simulink model "PV_module_model"  (R2022b)
settings: Solver=VariableStepAuto  StartTime=0.0  StopTime=1  FixedStep=10e-6  RelTol=1e-3
undefined symbols (not defined in the file): sigbuilder_block
libraries: slpidlib x1
settings Model: Creator=amahe  LastModifiedBy=amahe

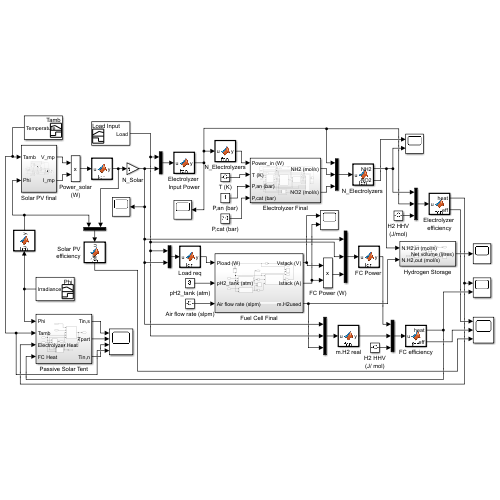
[thumbnail: Simulink's stored preview of the top-level diagram]
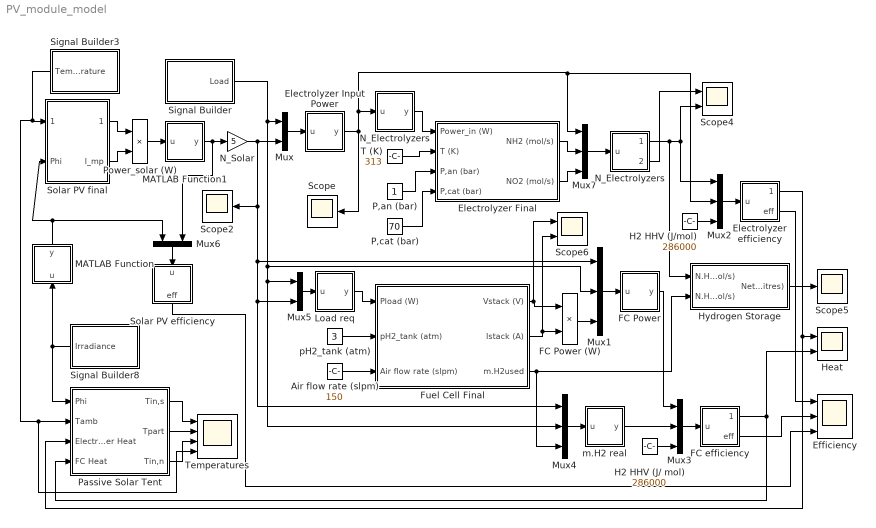
== system PV_module_model ==
  Air flow rate (slpm) : Constant  Value=150
  Efficiency : Scope  NumInputPorts=3
  Electrolyzer Input Power : MATLAB Function  TreatAsAtomicUnit=on
  Electrolyzer efficiency : MATLAB Function  TreatAsAtomicUnit=on
  Electrolyzer Final : Subsystem
  "FC Power " : MATLAB Function  TreatAsAtomicUnit=on
  FC Power (W) : Product
  FC efficiency : MATLAB Function  TreatAsAtomicUnit=on
  Fuel Cell Final : Subsystem
  H2 HHV (J/ mol) : Constant  Value=286000
  H2 HHV (J/mol) : Constant  Value=286000
  Heat : Scope  NumInputPorts=2
  Hydrogen Storage : Subsystem
  Load req : MATLAB Function  TreatAsAtomicUnit=on
  MATLAB Function : MATLAB Function  TreatAsAtomicUnit=on
  MATLAB Function1 : MATLAB Function  TreatAsAtomicUnit=on
  Mux : Mux  Inputs=2
  Mux{1..4,7} (5 alike) : Mux  Inputs=3
  Mux5 : Mux  Inputs=2
  Mux6 : Mux  Inputs=2
  N_Electrolyzers : MATLAB Function  TreatAsAtomicUnit=on
  "N_Electrolyzers " : MATLAB Function  TreatAsAtomicUnit=on
  N_Solar : Gain  Gain=5
  P,an (bar) : Constant
  P,cat (bar) : Constant  Value=70
  Passive Solar Tent : Subsystem
  Power_solar (W) : Product
  Scope : Scope
  Scope2 : Scope
  Scope4 : Scope  NumInputPorts=2
  Scope5 : Scope
  Scope6 : Scope  NumInputPorts=2
  Signal Builder : Subsystem  Tag=STV Subsys  LoadFcn=sigbuilder_block('load');  StartFcn=sigbuilder_block('start');  StopFcn=sigbuilder_block('stop');  ClipboardFcn=sigbuilder_block('clipboard');  mask(Sigbuilder block){tuvar=[0:10]}
      mask help: Simulink:masks:SigbuilderBlock_MD
      mask init:
      | if ~strcmp(get_param(bdroot(gcbh),'SimulationStatus'),'stopped') tuvar = sigbuilder_block('maskInit'); end
      settings: CopyFcn=sigbuilder_block('copy');  DeleteFcn=sigbuilder_block('delete');  ModelCloseFcn=sigbuilder_block('modelClose');  PreSaveFcn=sigbuilder_block('preSave');  PauseFcn=sigbuilder_block('pause');  ContinueFcn=sigbuilder_block('continue');  NameChangeFcn=sigbuilder_block('namechange');  OpenFcn=sigbuilder_block('open',[425.4 150.6 550.8 400.2 ]);  CloseFcn=sigbuilder_block('close');
      mask Display: plot(0, 0, 100, 100,[2, 2, 32, 32, 2], [68, 8, 8, 68, 68],[32, 2], [38, 38], [32, 19, 2],[53, 60, 44], [32, 17, 17, 2],[16, 16, 31, 31]);txt = getActiveGroup(gcbh);text(2, 100, txt,'verticalAlignment', 'top');
  Signal Builder3 : Subsystem  Tag=STV Subsys  LoadFcn=sigbuilder_block('load');  StartFcn=sigbuilder_block('start');  StopFcn=sigbuilder_block('stop');  ClipboardFcn=sigbuilder_block('clipboard');  mask(Sigbuilder block){tuvar=[0:10]}
      mask help: Simulink:masks:SigbuilderBlock_MD
      mask init:
      | if ~strcmp(get_param(bdroot(gcbh),'SimulationStatus'),'stopped') tuvar = sigbuilder_block('maskInit'); end
      settings: CopyFcn=sigbuilder_block('copy');  DeleteFcn=sigbuilder_block('delete');  ModelCloseFcn=sigbuilder_block('modelClose');  PreSaveFcn=sigbuilder_block('preSave');  PauseFcn=sigbuilder_block('pause');  ContinueFcn=sigbuilder_block('continue');  NameChangeFcn=sigbuilder_block('namechange');  OpenFcn=sigbuilder_block('open',[437.6 199.2 550.4 400 ]);  CloseFcn=sigbuilder_block('close');
      mask Display: plot(0, 0, 100, 100,[2, 2, 32, 32, 2], [68, 8, 8, 68, 68],[32, 2], [38, 38], [32, 19, 2],[53, 60, 44], [32, 17, 17, 2],[16, 16, 31, 31]);txt = getActiveGroup(gcbh);text(2, 100, txt,'verticalAlignment', 'top');
  Signal Builder8 : Subsystem  Tag=STV Subsys  LoadFcn=sigbuilder_block('load');  StartFcn=sigbuilder_block('start');  StopFcn=sigbuilder_block('stop');  ClipboardFcn=sigbuilder_block('clipboard');  mask(Sigbuilder block){tuvar=[0:10]}
      mask help: Simulink:masks:SigbuilderBlock_MD
      mask init:
      | if ~strcmp(get_param(bdroot(gcbh),'SimulationStatus'),'stopped') tuvar = sigbuilder_block('maskInit'); end
      settings: CopyFcn=sigbuilder_block('copy');  DeleteFcn=sigbuilder_block('delete');  ModelCloseFcn=sigbuilder_block('modelClose');  PreSaveFcn=sigbuilder_block('preSave');  PauseFcn=sigbuilder_block('pause');  ContinueFcn=sigbuilder_block('continue');  NameChangeFcn=sigbuilder_block('namechange');  OpenFcn=sigbuilder_block('open',[437.6 199.2 550.4 400 ]);  CloseFcn=sigbuilder_block('close');
      mask Display: plot(0, 0, 100, 100,[2, 2, 32, 32, 2], [68, 8, 8, 68, 68],[32, 2], [38, 38], [32, 19, 2],[53, 60, 44], [32, 17, 17, 2],[16, 16, 31, 31]);txt = getActiveGroup(gcbh);text(2, 100, txt,'verticalAlignment', 'top');
  Solar PV efficiency : MATLAB Function  TreatAsAtomicUnit=on
  Solar PV final : Subsystem
  T (K) : Constant  Value=313
  Temperatures : Scope  NumInputPorts=4
  m.H2 real : MATLAB Function  TreatAsAtomicUnit=on
  pH2_tank (atm) : Constant  Value=3
  wires:
  Electrolyzer Final/2(NO2 (mol/s)) -> Mux7/3
  Passive Solar Tent/1(Tin,s) -> Temperatures/1
  Mux7/1 -> "N_Electrolyzers "/1(u)
  Power_solar (W)/1 -> MATLAB Function1/1(u)
  "N_Electrolyzers "/1(NH2) -> Hydrogen Storage/1(N.H2,in (mol/s)), Mux2/1, Scope4/2
  FC efficiency/1(heat) -> Passive Solar Tent/4(FC Heat), Heat/2
  FC efficiency/2(eff) -> Efficiency/2
  Mux/1 -> Electrolyzer Input Power/1(u)
  P,cat (bar)/1 -> Electrolyzer Final/4(P,cat (bar))
  Mux6/1 -> Solar PV efficiency/1(u)
  Signal Builder3/1(Temperature) -> Passive Solar Tent/2(Tamb), Temperatures/4, Solar PV final/1(Tamb)
  Electrolyzer efficiency/1(heat) -> Passive Solar Tent/3(Electrolyzer Heat), Heat/1
  Air flow rate (slpm)/1 -> Fuel Cell Final/3(Air flow rate (slpm))
  m.H2 real/1(y) -> Mux3/2
  Electrolyzer efficiency/2(eff) -> Efficiency/1
  "N_Electrolyzers "/2(NO2) -> Scope4/1
  Hydrogen Storage/1(Net volume (litres)) -> Scope5/1
  Passive Solar Tent/2(Tpart) -> Temperatures/2
  Electrolyzer Input Power/1(y) -> Mux2/2, Mux7/1, N_Electrolyzers/1(u), Scope/1
  Mux3/1 -> FC efficiency/1(u)
  MATLAB Function/1(y) -> Mux6/1, Solar PV final/2(Phi)
  T (K)/1 -> Electrolyzer Final/2(T (K))
  FC Power (W)/1 -> Mux1/3
  Solar PV final/2(I_mp) -> Power_solar (W)/2
  Fuel Cell Final/2(Istack (A)) -> Scope6/2, FC Power (W)/2
  Fuel Cell Final/3(m.H2used) -> Mux4/3, Hydrogen Storage/2(N.H2,out (mol/s))
  Electrolyzer Final/1(NH2 (mol/s)) -> Mux7/2
  Passive Solar Tent/3(Tin,n) -> Temperatures/3
  Fuel Cell Final/1(Vstack (V)) -> Scope6/1, FC Power (W)/1
  MATLAB Function1/1(y) -> N_Solar/1, Mux6/2
  Mux2/1 -> Electrolyzer efficiency/1(u)
  Solar PV efficiency/1(eff) -> Efficiency/3
  Signal Builder/1(Load) -> Mux4/2, Mux5/1, Mux1/2, Mux/1
  P,an (bar)/1 -> Electrolyzer Final/3(P,an (bar))
  Mux1/1 -> "FC Power "/1(u)
  Signal Builder8/1(Irradiance) -> Passive Solar Tent/1(Phi), MATLAB Function/1(u)
  H2 HHV (J/ mol)/1 -> Mux3/3
  "FC Power "/1(y) -> Mux3/1
  pH2_tank (atm)/1 -> Fuel Cell Final/2(pH2_tank (atm))
  H2 HHV (J/mol)/1 -> Mux2/3
  Mux5/1 -> Load req/1(u)
  N_Electrolyzers/1(y) -> Electrolyzer Final/1(Power_in (W))
  Solar PV final/1(V_mp) -> Power_solar (W)/1
  Load req/1(y) -> Fuel Cell Final/1(Pload (W))
  N_Solar/1 -> Mux/2, Mux1/1, Mux4/1, Mux5/2, Scope2/1
  Mux4/1 -> m.H2 real/1(u)

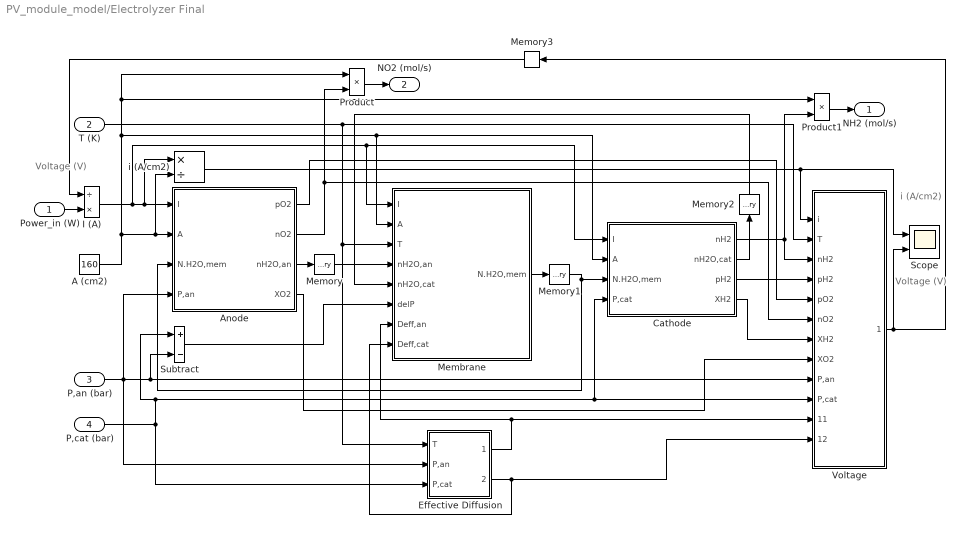
== system PV_module_model/Electrolyzer Final ==
  note: Voltage (V)
  note: i (A/cm2)
  note: Voltage
      | (V)
  Power_in (W) : Inport
  T (K) : Inport  Port=2
  P,an (bar) : Inport  Port=3
  P,cat (bar) : Inport  Port=4
  A (cm2) : Constant  Value=160
  Anode : Subsystem
  Cathode : Subsystem
  Effective Diffusion : Subsystem
  I (A) : Product  Inputs=/*
  Membrane : Subsystem
  Memory : Memory  InitialCondition=10^6
  Memory1 : Memory  InitialCondition=1
  Memory2 : Memory  InitialCondition=10^6
  Memory3 : Memory  InitialCondition=2
  Product : Product  Inputs=**
  Product1 : Product  Inputs=**
  Scope : Scope  NumInputPorts=2
  Subtract : Sum  Inputs=+-
  Voltage : Subsystem
  i (A/cm2) : Product  Inputs=*/
  NH2 (mol/s) : Outport
  NO2 (mol/s) : Outport  Port=2
  wires:
  A (cm2)/1 -> i (A/cm2)/2, Anode/2(A), Product/1, Product1/1, Cathode/2(A), Membrane/2(A)
  I (A)/1 -> Membrane/1(I), Cathode/1(I), i (A/cm2)/1, Anode/1(I)
  Cathode/3(pH2) -> Voltage/4(pH2)
  Membrane/1(N.H2O,mem) -> Memory1/1
  P,cat (bar)/1 -> Effective Diffusion/3(P,cat), Subtract/1, Cathode/4(P,cat), Voltage/10(P,cat)
  Anode/3(nH2O,an) -> Memory/1
  i (A/cm2)/1 -> Scope/1, Voltage/1(i)
  Memory/1 -> Membrane/4(nH2O,an)
  Anode/4(XO2) -> Voltage/8(XO2)
  Effective Diffusion/1(Deff,an) -> Voltage/11(Deff,an), Membrane/7(Deff,an)
  Voltage/1(Voltage (V)) -> Memory3/1, Scope/2
  Power_in (W)/1 -> I (A)/2
  T (K)/1 -> Membrane/3(T), Effective Diffusion/1(T), Voltage/2(T)
  Cathode/2(nH2O,cat) -> Memory2/1
  Memory1/1 -> Anode/3(N.H2O,mem), Cathode/3(N.H2O,mem)
  Memory2/1 -> Membrane/5(nH2O,cat)
  Memory3/1 -> I (A)/1
  Product/1 -> NO2 (mol/s)/1
  Effective Diffusion/2(Deff,cat) -> Voltage/12(Deff,cat), Membrane/8(Deff,cat)
  Cathode/4(XH2) -> Voltage/7(XH2)
  Cathode/1(nH2) -> Product1/2, Voltage/3(nH2)
  Subtract/1 -> Membrane/6(delP)
  Product1/1 -> NH2 (mol/s)/1
  Anode/1(pO2) -> Voltage/5(pO2)
  P,an (bar)/1 -> Anode/4(P,an), Effective Diffusion/2(P,an), Subtract/2, Voltage/9(P,an)
  Anode/2(nO2) -> Product/2, Voltage/6(nO2)

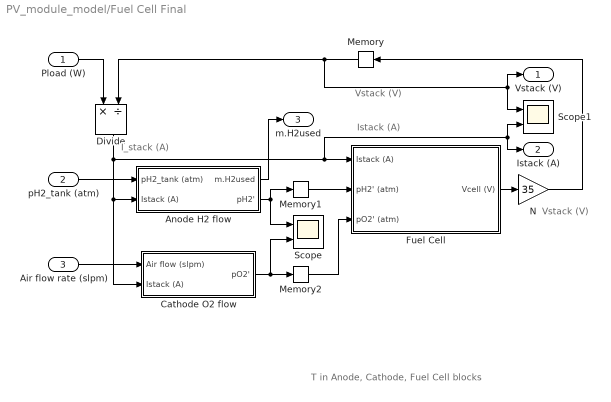
== system PV_module_model/Fuel Cell Final ==
  note: T in Anode, Cathode, Fuel Cell blocks
  note: I_stack (A)
  note: Vstack (V)
  note: Istack (A)
  note: Vstack (V)
  Pload (W) : Inport
  pH2_tank (atm) : Inport  Port=2
  Air flow rate (slpm) : Inport  Port=3
  Anode H2 flow : Subsystem
  Cathode O2 flow : Subsystem
  Divide : Product  Inputs=*/
  Fuel Cell : Subsystem
  Memory : Memory  InitialCondition=45
  Memory1 : Memory  InitialCondition=5
  Memory2 : Memory  InitialCondition=5
  N : Gain  Gain=35
  Scope : Scope  NumInputPorts=2
  Scope1 : Scope  NumInputPorts=2
  Vstack (V) : Outport
  Istack (A) : Outport  Port=2
  m.H2used : Outport  Port=3
  wires:
  Anode H2 flow/2(pH2') -> Memory1/1, Scope/1
  Air flow rate (slpm)/1 -> Cathode O2 flow/1(Air flow (slpm))
  Cathode O2 flow/1(pO2') -> Memory2/1, Scope/2
  Fuel Cell/1(Vcell (V)) -> N/1
  N/1 -> Memory/1
  pH2_tank (atm)/1 -> Anode H2 flow/1(pH2_tank (atm))
  Memory/1 -> Scope1/1, Vstack (V)/1, Divide/2
  Memory1/1 -> Fuel Cell/2(pH2' (atm))
  Memory2/1 -> Fuel Cell/3(pO2' (atm))
  Pload (W)/1 -> Divide/1
  Divide/1 -> Fuel Cell/1(Istack (A)), Scope1/2, Istack (A)/1, Anode H2 flow/2(Istack (A)), Cathode O2 flow/2(Istack (A))
  Anode H2 flow/1(m.H2used) -> m.H2used/1

== system PV_module_model/Hydrogen Storage ==
  N.H2,in (mol/s) : Inport
  N.H2,out (mol/s) : Inport  Port=2
  Mass (kg) : Gain  Gain=0.002
  NH2 produced (mol) : Integrator
  NH2 used (mol) : Integrator
  NH2,net (mol) : Sum  Inputs=+-
  Scope2 : Scope
  Volume (std. litres) : Gain  Gain=8.314*273.15/10^5*1000
  Net volume (litres) : Outport
  wires:
  N.H2,out (mol/s)/1 -> NH2 used (mol)/1
  NH2 produced (mol)/1 -> NH2,net (mol)/1
  NH2,net (mol)/1 -> Volume (std. litres)/1, Mass (kg)/1
  Volume (std. litres)/1 -> Net volume (litres)/1
  NH2 used (mol)/1 -> NH2,net (mol)/2
  N.H2,in (mol/s)/1 -> NH2 produced (mol)/1
  Mass (kg)/1 -> Scope2/1

== system PV_module_model/Passive Solar Tent ==
  Phi : Inport
  Tamb : Inport  Port=2
  Electrolyzer Heat : Inport  Port=3
  FC Heat : Inport  Port=4
  Memory : Memory  InitialCondition=280
  Memory1 : Memory  InitialCondition=278
  North side : Subsystem
  Partition : Subsystem
  South side : Subsystem
  Tin,s : Outport
  Tpart : Outport  Port=2
  Tin,n : Outport  Port=3
  wires:
  Partition/1(Tpart) -> Tpart/1, Memory/1
  FC Heat/1 -> North side/2(FC Heat)
  Memory1/1 -> Partition/1(Tin,n)
  Tamb/1 -> Partition/2(Tamb), South side/2(Tamb), North side/5(Tamb)
  Memory/1 -> North side/3(Tpart)
  North side/1(Tin,n) -> Tin,n/1, Memory1/1
  Phi/1 -> Partition/3(Phi), South side/1(Phi), North side/4(Phi)
  Electrolyzer Heat/1 -> North side/1(Electrolyzer Heat)
  South side/1(Tin,s) -> Tin,s/1

== system PV_module_model/Signal Builder ==
  Demux : Demux  Tag=STV Demux  Outputs=1
      settings: DisplayOption=none
  FromWs : FromWorkspace  Tag=STV FromWs  VariableName=tuvar
      SigBuilderData=|
      | common.afterFinalStr = 'Extrapolate'
      | common.sampleTime = 0
      | dataSet.timeRange = [0 1]
      | dataSet.name = 'Load Input'
      | sbobj.Groups.Name = 'Load Input'
      | sbobj.Groups.Signals.Name = 'Load'
      | sbobj.Groups.Signals.XData = [0 0.0105263157895 0.0210526315789 0.0315789473684 0.0421052631579 0.0526315789474 0.0631578947368 0.0736842105263 0.0842105263158 0.0947368421053 0.105263157895 0.115789473684 0.126315789474 0.136842105263 0.147368421053 0.157894736842 0.168421052632 0.178947368421 0.189473684211 0.2 0.210526315789 0.221052631579 0.231578947368 0.242105263158 0.252631578947 0.263157894737 0.273684210526 0.284210526316 0.294736842105 0.305263157895 0.315789473684 0.326315789474 0.336842105263 0.347368421053 0.357894736842 0.368421052632 0.378947368421 0.389473684211 0.4 0.410526315789 0.421052631579 0.431578947368 0.442105263158 0.452631578947 0.463157894737 0.473684210526 0.484210526316 0.494736842105 0.505263157895 0.515789473684 0.526315789474 0.536842105263 0.547368421053 0.557894736842 0.568421052632 0.578947368421 0.589473684211 0.6 0.610526315789 0.621052631579 0.631578947368 0.642105263158 0.652631578947 0.663157894737 0.673684210526 0.684210526316 0.694736842105 0.705263157895 0.715789473684 0.726315789474 0.736842105263 0.747368421053 0.757894736842 0.768421052632 0.778947368421 0.789473684211 0.8 0.810526315789 0.821052631579 0.831578947368 0.842105263158 0.852631578947 0.863157894737 0.873684210526 0.884210526316 0.894736842105 0.905263157895 0.915789473684 0.926315789474 0.936842105263 0.947368421053 0.957894736842 0.968421052632 0.978947368421 0.989473684211 1]
      | sbobj.Groups.Signals.YData = [410 390 350 335 320 325 325 330 335 335 340 345 350 355 365 370 350 345 340 360 370 385 400 415 430 460 485 500 510 525 535 550 560 540 520 500 480 450 410 340 320 305 265 225 210 195 170 135 105 90 65 40 15 5 15 30 35 25 20 15 10 20 40 75 115 165 190 225 260 335 400 470 580 665 750 770 805 845 870 905 935 955 970 925 910 870 815 780 750 670 610 570 495 440 400 370]
      | sbobj.Groups.TimeRange = [0 1]
  Load : Outport  Tag=STV Outport
  wires:
  Demux/1 -> Load/1
  FromWs/1 -> Demux/1

== system PV_module_model/Signal Builder3 ==
  Demux : Demux  Tag=STV Demux  Outputs=1
      settings: DisplayOption=none
  FromWs : FromWorkspace  Tag=STV FromWs  VariableName=tuvar
      SigBuilderData=|
      | common.afterFinalStr = 'Extrapolate'
      | common.sampleTime = 0
      | dataSet(1).timeRange = [0 1]
      | dataSet(1).name = 'Phi'
      | dataSet(2).timeRange = [0 1]
      | dataSet(2).name = 'Tamb'
      | dataSet(3).timeRange = [0 1]
      | dataSet(3).name = 'Tpart'
      | dataSet(4).timeRange = [0 1]
      | dataSet(4).name = 'Electrolyzer'
      | dataSet(5).timeRange = [0 1]
      | dataSet(5).name = 'Fuel Cell'
      | sbobj.Groups(1).Name = 'Phi'
      | sbobj.Groups(1).Signals.Name = 'Temperature'
      | sbobj.Groups(1).Signals.XData = [0 0.0105263157895 0.0210526315789 0.0315789473684 0.0421052631579 0.0526315789474 0.0631578947368 0.0736842105263 0.0842105263158 0.0947368421053 0.105263157895 0.115789473684 0.126315789474 0.136842105263 0.147368421053 0.157894736842 0.168421052632 0.178947368421 0.189473684211 0.2 0.210526315789 0.221052631579 0.231578947368 0.242105263158 0.252631578947 0.263157894737 0.273684210526 0.284210526316 0.294736842105 0.305263157895 0.315789473684 0.326315789474 0.336842105263 0.347368421053 0.357894736842 0.368421052632 0.378947368421 0.389473684211 0.4 0.410526315789 0.421052631579 0.431578947368 0.442105263158 0.452631578947 0.463157894737 0.473684210526 0.484210526316 0.494736842105 0.505263157895 0.515789473684 0.526315789474 0.536842105263 0.547368421053 0.557894736842 0.568421052632 0.578947368421 0.589473684211 0.6 0.610526315789 0.621052631579 0.631578947368 0.642105263158 0.652631578947 0.663157894737 0.673684210526 0.684210526316 0.694736842105 0.705263157895 0.715789473684 0.726315789474 0.736842105263 0.747368421053 0.757894736842 0.768421052632 0.778947368421 0.789473684211 0.8 0.810526315789 0.821052631579 0.831578947368 0.842105263158 0.852631578947 0.863157894737 0.873684210526 0.884210526316 0.894736842105 0.905263157895 0.915789473684 0.926315789474 0.936842105263 0.947368421053 0.957894736842 0.968421052632 0.978947368421 0.989473684211 1]
      | sbobj.Groups(1).Signals.YData = [0 0 0 0 0 0 0 0 0 0 0 0 0 0 0 0 0 0 0 0 0 0 112 161 213 266 321 378 433 488 542 595 646 695 742 788 831 870 907 942 972 999 1022 1043 1059 1071 1078 1083 1083 1078 1070 1059 1043 1023 999 970 939 905 868 829 786 741 694 645 594 541 487 433 378 322 267 214 162 112 0 0 0 0 0 0 0 0 0 0 0 0 0 0 0 0 0 0 0 0 0 0]
      | sbobj.Groups(1).TimeRange = [0 1]
      | sbobj.Groups(2).Name = 'Tamb'
      | sbobj.Groups(2).Signals.Name = 'Temperature'
      | sbobj.Groups(2).Signals.XData = [0 0.0105263157895 0.0210526315789 0.0315789473684 0.0421052631579 0.0526315789474 0.0631578947368 0.0736842105263 0.0842105263158 0.0947368421053 0.105263157895 0.115789473684 0.126315789474 0.136842105263 0.147368421053 0.157894736842 0.168421052632 0.178947368421 0.189473684211 0.2 0.210526315789 0.221052631579 0.231578947368 0.242105263158 0.252631578947 0.263157894737 0.273684210526 0.284210526316 0.294736842105 0.305263157895 0.315789473684 0.326315789474 0.336842105263 0.347368421053 0.357894736842 0.368421052632 0.378947368421 0.389473684211 0.4 0.410526315789 0.421052631579 0.431578947368 0.442105263158 0.452631578947 0.463157894737 0.473684210526 0.484210526316 0.494736842105 0.505263157895 0.515789473684 0.526315789474 0.536842105263 0.547368421053 0.557894736842 0.568421052632 0.578947368421 0.589473684211 0.6 0.610526315789 0.621052631579 0.631578947368 0.642105263158 0.652631578947 0.663157894737 0.673684210526 0.684210526316 0.694736842105 0.705263157895 0.715789473684 0.726315789474 0.736842105263 0.747368421053 0.757894736842 0.768421052632 0.778947368421 0.789473684211 0.8 0.810526315789 0.821052631579 0.831578947368 0.842105263158 0.852631578947 0.863157894737 0.873684210526 0.884210526316 0.894736842105 0.905263157895 0.915789473684 0.926315789474 0.936842105263 0.947368421053 0.957894736842 0.968421052632 0.978947368421 0.989473684211 1]
      | sbobj.Groups(2).Signals.YData = [277 277 276.9 276.9 276.8 276.8 276.8 276.7 276.7 276.7 276.7 276.7 276.7 276.7 276.7 276.7 276.7 276.7 276.7 276.7 277.5 278 278.6 279.1 279.7 280.2 280.7 281.2 281.7 282 282.4 282.7 283.1 283.4 283.6 283.9 284.2 284.4 284.7 284.9 285.1 285.3 285.4 285.6 285.7 285.8 285.9 286 286.1 286.1 286.1 286.1 286.2 286.1 286 286 285.9 285.8 285.6 285.5 285.4 285.2 285 284.8 284.6 284.4 284.1 283.9 283.7 283.4 283.1 282.8 282.6 282.2 281.9 281.6 281.3 281.1 281 280.9 280.8 280.7 280.6 280.4 280.3 280.2 280.1 280 279.8 279.7 279.6 279.5 279.4 279.2 279.1 279]
      | sbobj.Groups(2).TimeRange = [0 1]
      | sbobj.Groups(3).Name = 'Tpart'
      | sbobj.Groups(3).Signals.Name = 'Temperature'
      | sbobj.Groups(3).Signals.XData = [0 0.0105263157895 0.0210526315789 0.0315789473684 0.0421052631579 0.0526315789474 0.0631578947368 0.0736842105263 0.0842105263158 0.0947368421053 0.105263157895 0.115789473684 0.126315789474 0.136842105263 0.147368421053 0.157894736842 0.168421052632 0.178947368421 0.189473684211 0.2 0.210526315789 0.221052631579 0.231578947368 0.242105263158 0.252631578947 0.263157894737 0.273684210526 0.284210526316 0.294736842105 0.305263157895 0.315789473684 0.326315789474 0.336842105263 0.347368421053 0.357894736842 0.368421052632 0.378947368421 0.389473684211 0.4 0.410526315789 0.421052631579 0.431578947368 0.442105263158 0.452631578947 0.463157894737 0.473684210526 0.484210526316 0.494736842105 0.505263157895 0.515789473684 0.526315789474 0.536842105263 0.547368421053 0.557894736842 0.568421052632 0.578947368421 0.589473684211 0.6 0.610526315789 0.621052631579 0.631578947368 0.642105263158 0.652631578947 0.663157894737 0.673684210526 0.684210526316 0.694736842105 0.705263157895 0.715789473684 0.726315789474 0.736842105263 0.747368421053 0.757894736842 0.768421052632 0.778947368421 0.789473684211 0.8 0.810526315789 0.821052631579 0.831578947368 0.842105263158 0.852631578947 0.863157894737 0.873684210526 0.884210526316 0.894736842105 0.905263157895 0.915789473684 0.926315789474 0.936842105263 0.947368421053 0.957894736842 0.968421052632 0.978947368421 0.989473684211 1]
      | sbobj.Groups(3).Signals.YData = [297 297 296.9 296.9 296.8 296.8 296.8 296.7 296.7 296.7 296.7 296.7 296.7 296.7 296.7 296.7 296.7 296.7 296.7 296.7 297.5 298 298.6 299.1 299.7 300.2 300.7 301.2 301.7 302 302.4 302.7 303.1 303.4 303.6 303.9 304.2 304.4 304.7 304.9 305.1 305.3 305.4 305.6 305.7 305.8 305.9 306 306.1 306.1 306.1 306.1 306.2 306.1 306 306 305.9 305.8 305.6 305.5 305.4 305.2 305 304.8 304.6 304.4 304.1 303.9 303.7 303.4 303.1 302.8 302.6 302.2 301.9 301.6 301.3 301.1 301 300.9 300.8 300.7 300.6 300.4 300.3 300.2 300.1 300 299.8 299.7 299.6 299.5 299.4 299.2 299.1 299]
      | sbobj.Groups(3).TimeRange = [0 1]
      | sbobj.Groups(4).Name = 'Electrolyzer'
      | sbobj.Groups(4).Signals.Name = 'Temperature'
      | sbobj.Groups(4).Signals.XData = [0 5.52513948516e-06 1.10502789703e-05 1.65754184555e-05 2.21005579406e-05 2.76256974258e-05 3.3150836911e-05 3.86759763961e-05 4.42011158813e-05 4.97262553665e-05 5.52513948516e-05 6.07765343368e-05 ... (181221 elements, 1x181221)]
      | sbobj.Groups(4).Signals.YData = [0 0 0 0 0 0 0 0 0 0 0 0 ... (181221 elements, 1x181221)]
      | sbobj.Groups(4).TimeRange = [0 1]
      | sbobj.Groups(5).Name = 'Fuel Cell'
      | sbobj.Groups(5).Signals.Name = 'Temperature'
      | sbobj.Groups(5).Signals.XData = [0 5.52513948516e-06 1.10502789703e-05 1.65754184555e-05 2.21005579406e-05 2.76256974258e-05 3.3150836911e-05 3.86759763961e-05 4.42011158813e-05 4.97262553665e-05 5.52513948516e-05 6.07765343368e-05 ... (181221 elements, 1x181221)]
      | sbobj.Groups(5).Signals.YData = [61.8601336995 88.3587868316 0 193.960838345 190.648750401 185.476542263 181.849736228 179.072599417 176.825805801 174.941335652 173.319939397 171.898125993 ... (181221 elements, 1x181221)]
      | sbobj.Groups(5).TimeRange = [0 1]
  Temperature : Outport  Tag=STV Outport
  wires:
  Demux/1 -> Temperature/1
  FromWs/1 -> Demux/1

== system PV_module_model/Signal Builder8 ==
  Demux : Demux  Tag=STV Demux  Outputs=1
      settings: DisplayOption=none
  FromWs : FromWorkspace  Tag=STV FromWs  VariableName=tuvar
      SigBuilderData=|
      | common.afterFinalStr = 'Extrapolate'
      | common.sampleTime = 0
      | dataSet(1).timeRange = [0 1]
      | dataSet(1).name = 'Phi'
      | dataSet(2).timeRange = [0 1]
      | dataSet(2).name = 'Tamb'
      | dataSet(3).timeRange = [0 1]
      | dataSet(3).name = 'Tpart'
      | dataSet(4).timeRange = [0 1]
      | dataSet(4).name = 'Electrolyzer'
      | dataSet(5).timeRange = [0 1]
      | dataSet(5).name = 'Fuel Cell'
      | sbobj.Groups(1).Name = 'Phi'
      | sbobj.Groups(1).Signals.Name = 'Irradiance'
      | sbobj.Groups(1).Signals.XData = [0 0.0105263157895 0.0210526315789 0.0315789473684 0.0421052631579 0.0526315789474 0.0631578947368 0.0736842105263 0.0842105263158 0.0947368421053 0.105263157895 0.115789473684 0.126315789474 0.136842105263 0.147368421053 0.157894736842 0.168421052632 0.178947368421 0.189473684211 0.2 0.210526315789 0.221052631579 0.231578947368 0.242105263158 0.252631578947 0.263157894737 0.273684210526 0.284210526316 0.294736842105 0.305263157895 0.315789473684 0.326315789474 0.336842105263 0.347368421053 0.357894736842 0.368421052632 0.378947368421 0.389473684211 0.4 0.410526315789 0.421052631579 0.431578947368 0.442105263158 0.452631578947 0.463157894737 0.473684210526 0.484210526316 0.494736842105 0.505263157895 0.515789473684 0.526315789474 0.536842105263 0.547368421053 0.557894736842 0.568421052632 0.578947368421 0.589473684211 0.6 0.610526315789 0.621052631579 0.631578947368 0.642105263158 0.652631578947 0.663157894737 0.673684210526 0.684210526316 0.694736842105 0.705263157895 0.715789473684 0.726315789474 0.736842105263 0.747368421053 0.757894736842 0.768421052632 0.778947368421 0.789473684211 0.8 0.810526315789 0.821052631579 0.831578947368 0.842105263158 0.852631578947 0.863157894737 0.873684210526 0.884210526316 0.894736842105 0.905263157895 0.915789473684 0.926315789474 0.936842105263 0.947368421053 0.957894736842 0.968421052632 0.978947368421 0.989473684211 1]
      | sbobj.Groups(1).Signals.YData = [0 0 0 0 0 0 0 0 0 0 0 0 0 0 0 0 0 0 0 0 0 0 112 161 213 266 321 378 433 488 542 595 646 695 742 788 831 870 907 942 972 999 1022 1043 1059 1071 1078 1083 1083 1078 1070 1059 1043 1023 999 970 939 905 868 829 786 741 694 645 594 541 487 433 378 322 267 214 162 112 0 0 0 0 0 0 0 0 0 0 0 0 0 0 0 0 0 0 0 0 0 0]
      | sbobj.Groups(1).TimeRange = [0 1]
      | sbobj.Groups(2).Name = 'Tamb'
      | sbobj.Groups(2).Signals.Name = 'Irradiance'
      | sbobj.Groups(2).Signals.XData = [0 0.0105263157895 0.0210526315789 0.0315789473684 0.0421052631579 0.0526315789474 0.0631578947368 0.0736842105263 0.0842105263158 0.0947368421053 0.105263157895 0.115789473684 0.126315789474 0.136842105263 0.147368421053 0.157894736842 0.168421052632 0.178947368421 0.189473684211 0.2 0.210526315789 0.221052631579 0.231578947368 0.242105263158 0.252631578947 0.263157894737 0.273684210526 0.284210526316 0.294736842105 0.305263157895 0.315789473684 0.326315789474 0.336842105263 0.347368421053 0.357894736842 0.368421052632 0.378947368421 0.389473684211 0.4 0.410526315789 0.421052631579 0.431578947368 0.442105263158 0.452631578947 0.463157894737 0.473684210526 0.484210526316 0.494736842105 0.505263157895 0.515789473684 0.526315789474 0.536842105263 0.547368421053 0.557894736842 0.568421052632 0.578947368421 0.589473684211 0.6 0.610526315789 0.621052631579 0.631578947368 0.642105263158 0.652631578947 0.663157894737 0.673684210526 0.684210526316 0.694736842105 0.705263157895 0.715789473684 0.726315789474 0.736842105263 0.747368421053 0.757894736842 0.768421052632 0.778947368421 0.789473684211 0.8 0.810526315789 0.821052631579 0.831578947368 0.842105263158 0.852631578947 0.863157894737 0.873684210526 0.884210526316 0.894736842105 0.905263157895 0.915789473684 0.926315789474 0.936842105263 0.947368421053 0.957894736842 0.968421052632 0.978947368421 0.989473684211 1]
      | sbobj.Groups(2).Signals.YData = [277 277 276.9 276.9 276.8 276.8 276.8 276.7 276.7 276.7 276.7 276.7 276.7 276.7 276.7 276.7 276.7 276.7 276.7 276.7 277.5 278 278.6 279.1 279.7 280.2 280.7 281.2 281.7 282 282.4 282.7 283.1 283.4 283.6 283.9 284.2 284.4 284.7 284.9 285.1 285.3 285.4 285.6 285.7 285.8 285.9 286 286.1 286.1 286.1 286.1 286.2 286.1 286 286 285.9 285.8 285.6 285.5 285.4 285.2 285 284.8 284.6 284.4 284.1 283.9 283.7 283.4 283.1 282.8 282.6 282.2 281.9 281.6 281.3 281.1 281 280.9 280.8 280.7 280.6 280.4 280.3 280.2 280.1 280 279.8 279.7 279.6 279.5 279.4 279.2 279.1 279]
      | sbobj.Groups(2).TimeRange = [0 1]
      | sbobj.Groups(3).Name = 'Tpart'
      | sbobj.Groups(3).Signals.Name = 'Irradiance'
      | sbobj.Groups(3).Signals.XData = [0 0.0105263157895 0.0210526315789 0.0315789473684 0.0421052631579 0.0526315789474 0.0631578947368 0.0736842105263 0.0842105263158 0.0947368421053 0.105263157895 0.115789473684 0.126315789474 0.136842105263 0.147368421053 0.157894736842 0.168421052632 0.178947368421 0.189473684211 0.2 0.210526315789 0.221052631579 0.231578947368 0.242105263158 0.252631578947 0.263157894737 0.273684210526 0.284210526316 0.294736842105 0.305263157895 0.315789473684 0.326315789474 0.336842105263 0.347368421053 0.357894736842 0.368421052632 0.378947368421 0.389473684211 0.4 0.410526315789 0.421052631579 0.431578947368 0.442105263158 0.452631578947 0.463157894737 0.473684210526 0.484210526316 0.494736842105 0.505263157895 0.515789473684 0.526315789474 0.536842105263 0.547368421053 0.557894736842 0.568421052632 0.578947368421 0.589473684211 0.6 0.610526315789 0.621052631579 0.631578947368 0.642105263158 0.652631578947 0.663157894737 0.673684210526 0.684210526316 0.694736842105 0.705263157895 0.715789473684 0.726315789474 0.736842105263 0.747368421053 0.757894736842 0.768421052632 0.778947368421 0.789473684211 0.8 0.810526315789 0.821052631579 0.831578947368 0.842105263158 0.852631578947 0.863157894737 0.873684210526 0.884210526316 0.894736842105 0.905263157895 0.915789473684 0.926315789474 0.936842105263 0.947368421053 0.957894736842 0.968421052632 0.978947368421 0.989473684211 1]
      | sbobj.Groups(3).Signals.YData = [297 297 296.9 296.9 296.8 296.8 296.8 296.7 296.7 296.7 296.7 296.7 296.7 296.7 296.7 296.7 296.7 296.7 296.7 296.7 297.5 298 298.6 299.1 299.7 300.2 300.7 301.2 301.7 302 302.4 302.7 303.1 303.4 303.6 303.9 304.2 304.4 304.7 304.9 305.1 305.3 305.4 305.6 305.7 305.8 305.9 306 306.1 306.1 306.1 306.1 306.2 306.1 306 306 305.9 305.8 305.6 305.5 305.4 305.2 305 304.8 304.6 304.4 304.1 303.9 303.7 303.4 303.1 302.8 302.6 302.2 301.9 301.6 301.3 301.1 301 300.9 300.8 300.7 300.6 300.4 300.3 300.2 300.1 300 299.8 299.7 299.6 299.5 299.4 299.2 299.1 299]
      | sbobj.Groups(3).TimeRange = [0 1]
      | sbobj.Groups(4).Name = 'Electrolyzer'
      | sbobj.Groups(4).Signals.Name = 'Irradiance'
      | sbobj.Groups(4).Signals.XData = [0 5.52513948516e-06 1.10502789703e-05 1.65754184555e-05 2.21005579406e-05 2.76256974258e-05 3.3150836911e-05 3.86759763961e-05 4.42011158813e-05 4.97262553665e-05 5.52513948516e-05 6.07765343368e-05 ... (181221 elements, 1x181221)]
      | sbobj.Groups(4).Signals.YData = [0 0 0 0 0 0 0 0 0 0 0 0 ... (181221 elements, 1x181221)]
      | sbobj.Groups(4).TimeRange = [0 1]
      | sbobj.Groups(5).Name = 'Fuel Cell'
      | sbobj.Groups(5).Signals.Name = 'Irradiance'
      | sbobj.Groups(5).Signals.XData = [0 5.52513948516e-06 1.10502789703e-05 1.65754184555e-05 2.21005579406e-05 2.76256974258e-05 3.3150836911e-05 3.86759763961e-05 4.42011158813e-05 4.97262553665e-05 5.52513948516e-05 6.07765343368e-05 ... (181221 elements, 1x181221)]
      | sbobj.Groups(5).Signals.YData = [61.8601336995 88.3587868316 0 193.960838345 190.648750401 185.476542263 181.849736228 179.072599417 176.825805801 174.941335652 173.319939397 171.898125993 ... (181221 elements, 1x181221)]
      | sbobj.Groups(5).TimeRange = [0 1]
  Irradiance : Outport  Tag=STV Outport
  wires:
  Demux/1 -> Irradiance/1
  FromWs/1 -> Demux/1

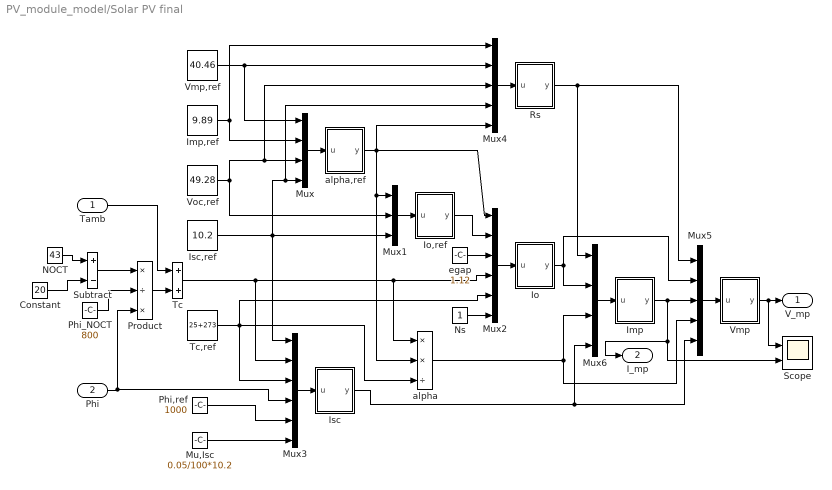
== system PV_module_model/Solar PV final ==
  Tamb : Inport
  Phi : Inport  Port=2
  Constant : Constant  Value=20
  Imp : MATLAB Function  TreatAsAtomicUnit=on
  Imp,ref : Constant  Value=9.89
  Io : MATLAB Function  TreatAsAtomicUnit=on
  Io,ref : MATLAB Function  TreatAsAtomicUnit=on
  Isc : MATLAB Function  TreatAsAtomicUnit=on
  Isc,ref : Constant  Value=10.2
  Mu,Isc : Constant  Value=0.05/100*10.2
  Mux : Mux
  Mux1 : Mux  Inputs=3
  Mux2 : Mux  Inputs=6
  Mux3 : Mux  Inputs=6
  Mux4 : Mux  Inputs=5
  Mux5 : Mux  Inputs=5
  Mux6 : Mux
  NOCT : Constant  Value=43
  Ns : Constant
  Phi,ref : Constant  Value=1000
  Phi_NOCT : Constant  Value=800
  Product : Product  Inputs=*/*
  Rs : MATLAB Function  TreatAsAtomicUnit=on
  Scope : Scope  NumInputPorts=2
  Subtract : Sum  Inputs=+-
  Tc : Sum
  Tc,ref : Constant  Value=25+273
  Vmp : MATLAB Function  TreatAsAtomicUnit=on
  Vmp,ref : Constant  Value=40.46
  Voc,ref : Constant  Value=49.28
  alpha : Product  Inputs=**/
  alpha,ref : MATLAB Function  TreatAsAtomicUnit=on
  egap : Constant  Value=1.12
  V_mp : Outport
  I_mp : Outport  Port=2
  wires:
  Mux/1 -> alpha,ref/1(u)
  Voc,ref/1 -> Mux1/2, Mux4/3, Mux/3
  alpha,ref/1(y) -> alpha/2, Mux1/1, Mux2/1, Mux4/5
  Isc,ref/1 -> Mux4/4, Mux/4, Mux1/3, Mux3/1
  Vmp,ref/1 -> Mux4/2, Mux/1
  Io,ref/1(y) -> Mux2/2
  Mux1/1 -> Io,ref/1(u)
  Mux4/1 -> Rs/1(u)
  Imp,ref/1 -> Mux/2, Mux4/1
  Tc/1 -> alpha/1, Mux2/4, Mux3/2
  Tc,ref/1 -> alpha/3, Mux2/5, Mux3/3
  Vmp/1(y) -> Scope/1, V_mp/1
  Mux5/1 -> Vmp/1(u)
  Phi,ref/1 -> Mux3/5
  Mux3/1 -> Isc/1(u)
  Mu,Isc/1 -> Mux3/6
  Ns/1 -> Mux2/6
  Phi/1 -> Product/3, Mux3/4
  Mux2/1 -> Io/1(u)
  egap/1 -> Mux2/3
  Isc/1(y) -> Mux5/5, Mux6/4
  alpha/1 -> Mux5/4, Mux6/3
  Io/1(y) -> Mux5/2, Mux6/2
  Rs/1(y) -> Mux5/1, Mux6/1
  Mux6/1 -> Imp/1(u)
  Imp/1(y) -> Mux5/3, Scope/2, I_mp/1
  NOCT/1 -> Subtract/1
  Constant/1 -> Subtract/2
  Subtract/1 -> Product/1
  Phi_NOCT/1 -> Product/2
  Product/1 -> Tc/2
  Tamb/1 -> Tc/1

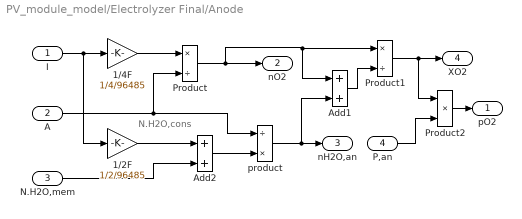
== system PV_module_model/Electrolyzer Final/Anode ==
  note: N.H2O,cons
  I : Inport
  A : Inport  Port=2
  N.H2O,mem : Inport  Port=3
  P,an : Inport  Port=4
  1/2F : Gain  Gain=1/2/96485
  1/4F : Gain  Gain=1/4/96485
  Add1 : Sum
  Add2 : Sum
  Product : Product  Inputs=*/
  Product1 : Product  Inputs=*/
  Product2 : Product  Inputs=**
  product : Product  Inputs=/*
  pO2 : Outport
  nO2 : Outport  Port=2
  nH2O,an : Outport  Port=3
  XO2 : Outport  Port=4
  wires:
  P,an/1 -> Product2/2
  Add2/1 -> product/2
  1/4F/1 -> Product/1
  Add1/1 -> Product1/2
  A/1 -> product/1, Product/2
  Product/1 -> nO2/1, Product1/1, Add1/1
  product/1 -> nH2O,an/1, Add1/2
  Product1/1 -> XO2/1, Product2/1
  I/1 -> 1/2F/1, 1/4F/1
  Product2/1 -> pO2/1
  1/2F/1 -> Add2/1
  N.H2O,mem/1 -> Add2/2

== system PV_module_model/Electrolyzer Final/Cathode ==
  I : Inport
  A : Inport  Port=2
  N.H2O,mem : Inport  Port=3
  P,cat : Inport  Port=4
  1/2F : Gain  Gain=1/2/96485
  Add1 : Sum
  Product : Product  Inputs=*/
  Product1 : Product  Inputs=*/
  Product2 : Product  Inputs=**
  product : Product  Inputs=/*
  nH2 : Outport
  nH2O,cat : Outport  Port=2
  pH2 : Outport  Port=3
  XH2 : Outport  Port=4
  wires:
  Product1/1 -> XH2/1, Product2/1
  A/1 -> product/1, Product/2
  Add1/1 -> Product1/2
  Product2/1 -> pH2/1
  Product/1 -> nH2/1, Product1/1, Add1/1
  I/1 -> 1/2F/1
  1/2F/1 -> Product/1
  P,cat/1 -> Product2/2
  product/1 -> nH2O,cat/1, Add1/2
  N.H2O,mem/1 -> product/2

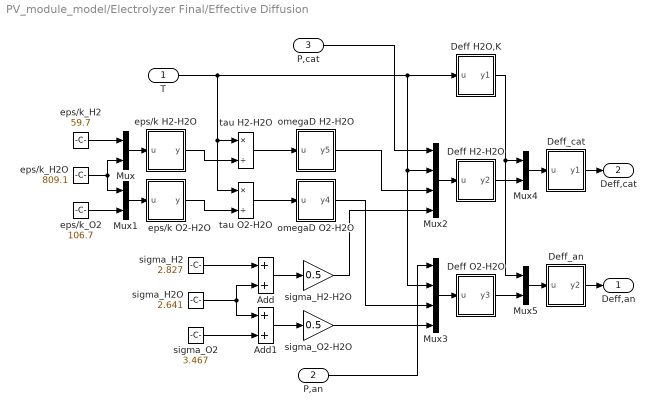
== system PV_module_model/Electrolyzer Final/Effective Diffusion ==
  T : Inport
  P,an : Inport  Port=2
  P,cat : Inport  Port=3
  Add : Sum
  Add1 : Sum
  Deff H2-H2O : MATLAB Function  TreatAsAtomicUnit=on
  Deff H2O,K : MATLAB Function  TreatAsAtomicUnit=on
  Deff O2-H2O : MATLAB Function  TreatAsAtomicUnit=on
  Deff_an : MATLAB Function  TreatAsAtomicUnit=on
  Deff_cat : MATLAB Function  TreatAsAtomicUnit=on
  Mux{,1,4..5} (4 alike) : Mux  Inputs=2
  Mux2 : Mux
  Mux3 : Mux
  eps/k H2-H2O : MATLAB Function  TreatAsAtomicUnit=on
  eps/k O2-H2O : MATLAB Function  TreatAsAtomicUnit=on
  eps/k_H2 : Constant  Value=59.7
  eps/k_H2O : Constant  Value=809.1
  eps/k_O2 : Constant  Value=106.7
  omegaD H2-H2O : MATLAB Function  TreatAsAtomicUnit=on
  omegaD O2-H2O : MATLAB Function  TreatAsAtomicUnit=on
  sigma_H2 : Constant  Value=2.827
  sigma_H2-H2O : Gain  Gain=0.5
  sigma_H2O : Constant  Value=2.641
  sigma_O2 : Constant  Value=3.467
  sigma_O2-H2O : Gain  Gain=0.5
  tau H2-H2O : Product  Inputs=*/
  tau O2-H2O : Product  Inputs=*/
  Deff,an : Outport
  Deff,cat : Outport  Port=2
  wires:
  Mux/1 -> eps/k H2-H2O/1(u)
  Deff H2O,K/1(y1) -> Mux4/1, Mux5/1
  Add1/1 -> sigma_O2-H2O/1
  Deff O2-H2O/1(y3) -> Mux5/2
  T/1 -> tau O2-H2O/1, tau H2-H2O/1, Deff H2O,K/1(u), Mux3/2, Mux2/2
  eps/k_H2O/1 -> Mux1/1, Mux/2
  tau O2-H2O/1 -> omegaD O2-H2O/1(u)
  eps/k_H2/1 -> Mux/1
  Add/1 -> sigma_H2-H2O/1
  Mux2/1 -> Deff H2-H2O/1(u)
  Deff_an/1(y2) -> Deff,an/1
  omegaD H2-H2O/1(y5) -> Mux2/3
  sigma_H2-H2O/1 -> Mux2/4
  Mux4/1 -> Deff_cat/1(u)
  omegaD O2-H2O/1(y4) -> Mux3/3
  tau H2-H2O/1 -> omegaD H2-H2O/1(u)
  sigma_H2O/1 -> Add1/1, Add/2
  Mux1/1 -> eps/k O2-H2O/1(u)
  Deff H2-H2O/1(y2) -> Mux4/2
  sigma_O2/1 -> Add1/2
  sigma_H2/1 -> Add/1
  eps/k O2-H2O/1(y) -> tau O2-H2O/2
  eps/k_O2/1 -> Mux1/2
  eps/k H2-H2O/1(y) -> tau H2-H2O/2
  Deff_cat/1(y1) -> Deff,cat/1
  P,cat/1 -> Mux2/1
  Mux5/1 -> Deff_an/1(u)
  P,an/1 -> Mux3/1
  sigma_O2-H2O/1 -> Mux3/4
  Mux3/1 -> Deff O2-H2O/1(u)

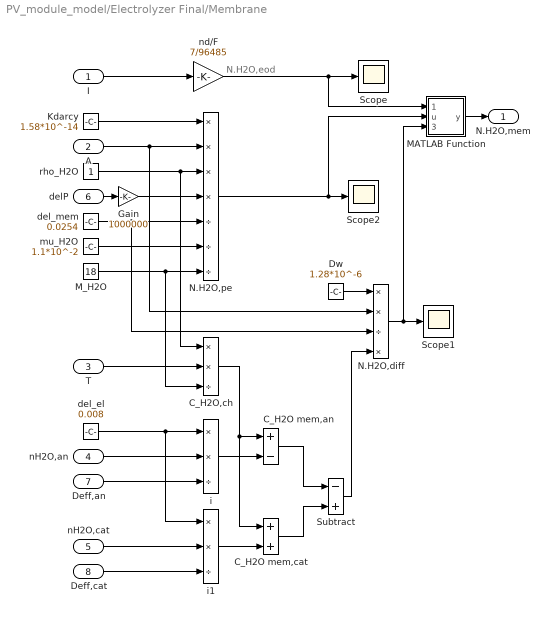
== system PV_module_model/Electrolyzer Final/Membrane ==
  note: N.H2O,eod
  I : Inport
  A : Inport  Port=2
  T : Inport  Port=3
  nH2O,an : Inport  Port=4
  nH2O,cat : Inport  Port=5
  delP : Inport  Port=6
  Deff,an : Inport  Port=7
  Deff,cat : Inport  Port=8
  C_H2O mem,an : Sum  Inputs=+-
  C_H2O mem,cat : Sum
  C_H2O,ch : Product  Inputs=**/
  Dw : Constant  Value=1.28*10^-6
  Gain : Gain  Gain=1000000
  Kdarcy : Constant  Value=1.58*10^-14
  MATLAB Function : MATLAB Function  TreatAsAtomicUnit=on
  M_H2O : Constant  Value=18
  N.H2O,diff : Product  Inputs=**/*
  N.H2O,pe : Product  Inputs=****///
  Scope : Scope
  Scope1 : Scope
  Scope2 : Scope
  Subtract : Sum  Inputs=-+
  del_el : Constant  Value=0.008
  del_mem : Constant  Value=0.0254
  i : Product  Inputs=**/
  i1 : Product  Inputs=**/
  mu_H2O : Constant  Value=1.1*10^-2
  nd/F : Gain  Gain=7/96485
  rho_H2O : Constant
  N.H2O,mem : Outport
  wires:
  M_H2O/1 -> C_H2O,ch/3, N.H2O,pe/7
  C_H2O mem,an/1 -> Subtract/1
  del_el/1 -> i1/1, i/1
  nd/F/1 -> MATLAB Function/1(data1), Scope/1
  Deff,cat/1 -> i1/3
  T/1 -> C_H2O,ch/2
  nH2O,an/1 -> i/2
  i/1 -> C_H2O mem,an/2
  C_H2O mem,cat/1 -> Subtract/2
  Dw/1 -> N.H2O,diff/1
  i1/1 -> C_H2O mem,cat/2
  Subtract/1 -> N.H2O,diff/4
  Kdarcy/1 -> N.H2O,pe/1
  I/1 -> nd/F/1
  C_H2O,ch/1 -> C_H2O mem,cat/1, C_H2O mem,an/1
  N.H2O,diff/1 -> MATLAB Function/3(data), Scope1/1
  A/1 -> N.H2O,diff/2, N.H2O,pe/2
  MATLAB Function/1(y) -> N.H2O,mem/1
  rho_H2O/1 -> C_H2O,ch/1, N.H2O,pe/3
  nH2O,cat/1 -> i1/2
  del_mem/1 -> N.H2O,pe/5, N.H2O,diff/3
  Deff,an/1 -> i/3
  N.H2O,pe/1 -> MATLAB Function/2(u), Scope2/1
  mu_H2O/1 -> N.H2O,pe/6
  delP/1 -> Gain/1
  Gain/1 -> N.H2O,pe/4

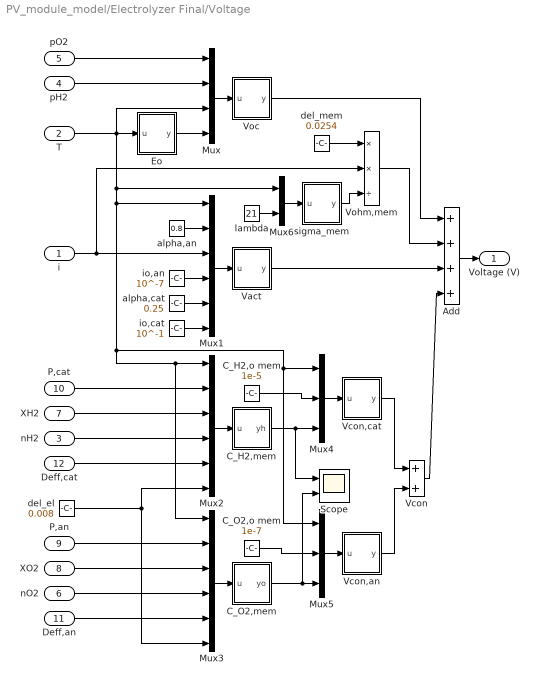
== system PV_module_model/Electrolyzer Final/Voltage ==
  i : Inport
  T : Inport  Port=2
  nH2 : Inport  Port=3
  pH2 : Inport  Port=4
  pO2 : Inport  Port=5
  nO2 : Inport  Port=6
  XH2 : Inport  Port=7
  XO2 : Inport  Port=8
  P,an : Inport  Port=9
  P,cat : Inport  Port=10
  Deff,an : Inport  Port=11
  Deff,cat : Inport  Port=12
  Add : Sum  Inputs=4
  C_H2,mem : MATLAB Function  TreatAsAtomicUnit=on
  C_H2,o mem : Constant  Value=1e-5
  C_O2,mem : MATLAB Function  TreatAsAtomicUnit=on
  C_O2,o mem : Constant  Value=1e-7
  Eo : MATLAB Function  TreatAsAtomicUnit=on
  Mux : Mux
  Mux1 : Mux  Inputs=6
  Mux2 : Mux  Inputs=6
  Mux3 : Mux  Inputs=6
  Mux4 : Mux  Inputs=3
  Mux5 : Mux  Inputs=3
  Mux6 : Mux  Inputs=2
  Scope : Scope  NumInputPorts=2
  Vact : MATLAB Function  TreatAsAtomicUnit=on
  Vcon : Sum
  Vcon,an : MATLAB Function  TreatAsAtomicUnit=on
  Vcon,cat : MATLAB Function  TreatAsAtomicUnit=on
  Voc : MATLAB Function  TreatAsAtomicUnit=on
  Vohm,mem : Product  Inputs=**/
  alpha,an : Constant  Value=0.8
  alpha,cat : Constant  Value=0.25
  del_el : Constant  Value=0.008
  del_mem : Constant  Value=0.0254
  io,an : Constant  Value=10^-7
  io,cat : Constant  Value=10^-1
  lambda : Constant  Value=21
  sigma_mem : MATLAB Function  TreatAsAtomicUnit=on
  Voltage (V) : Outport
  wires:
  XH2/1 -> Mux2/3
  T/1 -> Mux6/1, Mux5/1, Mux4/1, Mux3/1, Mux2/1, Mux1/1, Mux/3, Eo/1(u)
  nH2/1 -> Mux2/4
  C_O2,o mem/1 -> Mux5/2
  lambda/1 -> Mux6/2
  pH2/1 -> Mux/2
  Mux6/1 -> sigma_mem/1(u)
  pO2/1 -> Mux/1
  alpha,an/1 -> Mux1/2
  Voc/1(y) -> Add/1
  Mux/1 -> Voc/1(u)
  alpha,cat/1 -> Mux1/5
  Mux1/1 -> Vact/1(u)
  C_O2,mem/1(yo) -> Scope/2, Mux5/3
  Add/1 -> Voltage (V)/1
  del_el/1 -> Mux3/6, Mux2/6
  io,cat/1 -> Mux1/6
  Eo/1(y) -> Mux/4
  Vcon,cat/1(y) -> Vcon/1
  P,cat/1 -> Mux2/2
  nO2/1 -> Mux3/4
  sigma_mem/1(y) -> Vohm,mem/3
  Vohm,mem/1 -> Add/2
  Deff,cat/1 -> Mux2/5
  io,an/1 -> Mux1/4
  XO2/1 -> Mux3/3
  del_mem/1 -> Vohm,mem/1
  i/1 -> Mux1/3, Vohm,mem/2
  Vcon,an/1(y) -> Vcon/2
  Vact/1(y) -> Add/3
  Mux3/1 -> C_O2,mem/1(u)
  Mux4/1 -> Vcon,cat/1(u)
  Deff,an/1 -> Mux3/5
  P,an/1 -> Mux3/2
  Mux2/1 -> C_H2,mem/1(u)
  Mux5/1 -> Vcon,an/1(u)
  C_H2,o mem/1 -> Mux4/2
  C_H2,mem/1(yh) -> Scope/1, Mux4/3
  Vcon/1 -> Add/4

== system PV_module_model/Fuel Cell Final/Anode H2 flow ==
  note: m.H2out
  note: m.H2in
  pH2_tank (atm) : Inport
  Istack (A) : Inport  Port=2
  Memory4 : Memory  InitialCondition=0.1
  NI/2F : Gain  Gain=35/2/96485
  PID Controller : slpidlib/PID Controller  Controller=PID  Form=Parallel  TimeDomain=Continuous-time  UseExternalTs=off  SampleTime=-1  IntegratorMethod=Forward Euler  FilterMethod=Forward Euler  ControllerParametersSource=internal  P=1  I=1  UseKiTs=off  D=1  N=100  UseFilter=on  TunerSelectOption=Transfer Function Based (PID Tuner App)  InitialConditionSource=internal  InitialConditionForIntegrator=0  InitialConditionForFilter=0  DifferentiatorICPrevScaledInput=0  ExternalReset=none  TrackingMode=off  Kt=1  LimitOutput=off  SatLimitsSource=internal  UpperSaturationLimit=inf  LowerSaturationLimit=-inf  LinearizeAsGain=on  AntiWindupMode=none  Kb=1  LimitIntegrator=off  UpperIntegratorSaturationLimit=inf  LowerIntegratorSaturationLimit=-inf  POutMin=[]  POutMax=[]  IOutMin=[]  IOutMax=[]  DOutMin=[]  DOutMax=[]  NOutMin=[]  NOutMax=[]  SumOutMin=[]  SumOutMax=[]  SaturationOutMin=[]  SaturationOutMax=[]  PParamMin=[]  PParamMax=[]  IParamMin=[]  IParamMax=[]  DParamMin=[]  DParamMax=[]  NParamMin=[]  NParamMax=[]  KbParamMin=[]  KbParamMax=[]  KtParamMin=[]  KtParamMax=[]  KbOutMin=[]  KbOutMax=[]  KtOutMin=[]  KtOutMax=[]  IntegratorOutMin=[]  IntegratorOutMax=[]  FilterOutMin=[]  FilterOutMax=[]  SumI1OutMin=[]  SumI1OutMax=[]  SumI2OutMin=[]  SumI2OutMax=[]  SumI3OutMin=[]  SumI3OutMax=[]  SumI4OutMin=[]  SumI4OutMax=[]  SumDOutMin=[]  SumDOutMax=[]  DifferentiatorOutMin=[]  DifferentiatorOutMax=[]  FilterDiffOutCoefMin=[]  FilterDiffOutCoefMax=[]  ReciprocalOutMin=[]  ReciprocalOutMax=[]  SumDenOutMin=[]  SumDenOutMax=[]  SumNumOutMin=[]  SumNumOutMax=[]  DivideOutMin=[]  DivideOutMax=[]  UdiffTsProdOutMin=[]  UdiffTsProdOutMax=[]  NTsProdOutMin=[]  NTsProdOutMax=[]  UintegralTsProdOutMin=[]  UintegralTsProdOutMax=[]  UngainTsProdOutMin=[]  UngainTsProdOutMax=[]  ClampingZeroOutDataTypeStr=Inherit: Inherit via back propagation  ClampingZeroOutMin=[]  ClampingZeroOutMax=[]  FilterDenConstantOutDataTypeStr=Inherit: Inherit via back propagation  FilterDenConstantOutMin=[]  FilterDenConstantOutMax=[]  PCopyOutDataTypeStr=Inherit: Inherit via back propagation  PCopyOutMin=[]  PCopyOutMax=[]  NCopyOutDataTypeStr=Inherit: Inherit via back propagation  NCopyOutMin=[]  NCopyOutMax=[]  IntegratorContinuousStateAttributes=''  IntegratorStateMustResolveToSignalObject=off  IntegratorRTWStateStorageClass=Auto  FilterContinuousStateAttributes=''  FilterStateMustResolveToSignalObject=off  FilterRTWStateStorageClass=Auto  ParallelPVariant=InternalParameters  IdealPVariant=Disabled  IVariant=InternalParameters  DVariant=InternalParameters  IntegratorVariant=Continuous  SatVariant=Disabled  AWVariant=Passthrough  PCopyVariant=Disabled  TRVariant=Disabled  FdbkBlocksVariant=Forward  IdealPFdbkVariant=Disabled  SatFdbkVariant=Disabled  DerivativeFilterVariant=ContFilter  NVariant=InternalParameters  NCopyVariant=Disabled  FilterICVariant=InternalICsFilter  IntegratorICVariant=InternalICs  ExternalResetVariant=Disabled  TRSumVariant=Passthrough  SumFdbkVariant=Disabled  SumVariant=Sum_PID  TsampFilterVariant=InternalTs  TsampNgainVariant=Passthrough  TsampIntegralVariant=Passthrough  ExternalSaturationOutDataTypeStr=Inherit: Same as second input
  RT/Va : Gain  Gain=8.314*333/0.005/(1.013*10^5)
  Scope : Scope  NumInputPorts=4
  Subtract : Sum  Inputs=+--
  Sum : Sum  Inputs=|+-
  Sum1 : Sum  Inputs=|+-
  Transfer Fcn : TransferFcn  Denominator=[1 0]
  flow const : Gain  Gain=0.065
  flow_const : Gain  Gain=0.065
  m.H2used : Outport
  pH2' : Outport  Port=2
  wires:
  NI/2F/1 -> Scope/2, Subtract/2, m.H2used/1
  Transfer Fcn/1 -> Sum1/2, Sum/1, pH2'/1
  RT/Va/1 -> Transfer Fcn/1
  Memory4/1 -> Scope/3, Subtract/3
  Istack (A)/1 -> NI/2F/1
  Sum1/1 -> PID Controller/1
  Sum/1 -> flow const/1
  PID Controller/1 -> flow_const/1
  flow_const/1 -> Scope/1, Subtract/1
  flow const/1 -> Memory4/1
  Subtract/1 -> Scope/4, RT/Va/1
  pH2_tank (atm)/1 -> Sum1/1, Sum/2

== system PV_module_model/Fuel Cell Final/Cathode O2 flow ==
  note: m.O2in
  note: m.O2out
  Air flow (slpm) : Inport
  Istack (A) : Inport  Port=2
  NI/4F : Gain  Gain=35/4/96485
  O2 mole frac : Gain  Gain=0.21
  Pbpr : Constant  Value=3
  RT/Vc : Gain  Gain=8.314*333/0.01/(1.013*10^5)
  Subtract : Sum  Inputs=+--
  Sum : Sum  Inputs=|+-
  Transfer Fcn : TransferFcn  Denominator=[1 0]
  flow const : Gain  Gain=0.065
  mole/sec : Gain  Gain=7.34e-4
  pO2' : Outport
  wires:
  RT/Vc/1 -> Transfer Fcn/1
  Istack (A)/1 -> NI/4F/1
  flow const/1 -> Subtract/3
  Subtract/1 -> RT/Vc/1
  mole/sec/1 -> O2 mole frac/1
  Sum/1 -> flow const/1
  Pbpr/1 -> Sum/2
  Air flow (slpm)/1 -> mole/sec/1
  O2 mole frac/1 -> Subtract/1
  NI/4F/1 -> Subtract/2
  Transfer Fcn/1 -> pO2'/1, Sum/1

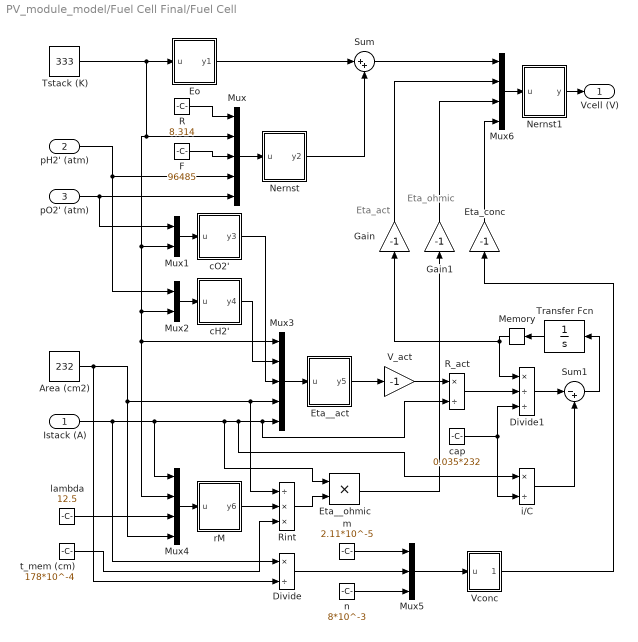
== system PV_module_model/Fuel Cell Final/Fuel Cell ==
  note: Eta_ohmic
  note: Eta_act
  Istack (A) : Inport
  pH2' (atm) : Inport  Port=2
  pO2' (atm) : Inport  Port=3
  Area (cm2) : Constant  Value=232
  Divide : Product  Inputs=*/
  Divide1 : Product  Inputs=*//
  Eo : MATLAB Function  TreatAsAtomicUnit=on
  Eta__act : MATLAB Function  TreatAsAtomicUnit=on
  Eta__ohmic : Product
  Eta_conc : Gain  Gain=-1
  F : Constant  Value=96485
  Gain : Gain  Gain=-1
  Gain1 : Gain  Gain=-1
  Memory : Memory  InitialCondition=0.01
  Mux : Mux  Inputs=5
  Mux1 : Mux  Inputs=2
  Mux2 : Mux  Inputs=2
  Mux3 : Mux  Inputs=5
  Mux4 : Mux
  Mux5 : Mux  Inputs=3
  Mux6 : Mux
  Nernst : MATLAB Function  TreatAsAtomicUnit=on
  Nernst1 : MATLAB Function  TreatAsAtomicUnit=on
  R : Constant  Value=8.314
  R_act : Product  Inputs=*/
  Rint : Product  Inputs=/**
  Sum : Sum  Inputs=|++
  Sum1 : Sum  Inputs=|-+
  Transfer Fcn : TransferFcn  Denominator=[1 0]
  Tstack (K) : Constant  Value=333
  V_act : Gain  Gain=-1
  Vconc : MATLAB Function  TreatAsAtomicUnit=on
  cH2' : MATLAB Function  TreatAsAtomicUnit=on
  cO2' : MATLAB Function  TreatAsAtomicUnit=on
  cap : Constant  Value=0.035*232
  i/C : Product  Inputs=*/
  lambda : Constant  Value=12.5
  m : Constant  Value=2.11*10^-5
  n : Constant  Value=8*10^-3
  rM : MATLAB Function  TreatAsAtomicUnit=on
  t_mem (cm) : Constant  Value=178*10^-4
  Vcell (V) : Outport
  wires:
  pO2' (atm)/1 -> Mux/5, Mux1/1
  Area (cm2)/1 -> Divide/2, Mux4/4, Rint/1, Mux3/4
  pH2' (atm)/1 -> Mux2/1, Mux/4
  Nernst1/1(y) -> Vcell (V)/1
  Mux/1 -> Nernst/1(u)
  Eo/1(y1) -> Sum/1
  Tstack (K)/1 -> Mux4/2, Mux3/1, Mux2/2, Mux1/2, Mux/2, Eo/1(u)
  cO2'/1(y3) -> Mux3/3
  m/1 -> Mux5/1
  R_act/1 -> Divide1/2
  F/1 -> Mux/3
  Mux1/1 -> cO2'/1(u)
  Nernst/1(y2) -> Sum/2
  Eta__ohmic/1 -> Gain1/1
  Sum1/1 -> Transfer Fcn/1
  Mux4/1 -> rM/1(u)
  Mux2/1 -> cH2'/1(u)
  Mux3/1 -> Eta__act/1(u)
  R/1 -> Mux/1
  Divide1/1 -> Sum1/1
  cap/1 -> i/C/2, Divide1/3
  t_mem (cm)/1 -> Rint/3
  cH2'/1(y4) -> Mux3/2
  Eta__act/1(y5) -> V_act/1
  Rint/1 -> Eta__ohmic/2
  i/C/1 -> Sum1/2
  V_act/1 -> R_act/1
  Transfer Fcn/1 -> Memory/1
  Mux5/1 -> Vconc/1(u)
  rM/1(y6) -> Rint/2
  n/1 -> Mux5/3
  Vconc/1(y7) -> Eta_conc/1
  lambda/1 -> Mux4/3
  Memory/1 -> Divide1/1, Gain/1
  Istack (A)/1 -> Divide/1, Mux4/1, Eta__ohmic/1, i/C/1, R_act/2, Mux3/5
  Divide/1 -> Mux5/2
  Mux6/1 -> Nernst1/1(u)
  Sum/1 -> Mux6/1
  Gain/1 -> Mux6/2
  Gain1/1 -> Mux6/3
  Eta_conc/1 -> Mux6/4

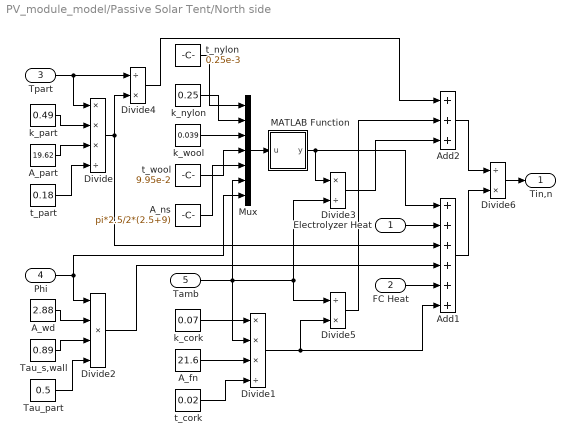
== system PV_module_model/Passive Solar Tent/North side ==
  Electrolyzer Heat : Inport
  FC Heat : Inport  Port=2
  Tpart : Inport  Port=3
  Phi : Inport  Port=4
  Tamb : Inport  Port=5
  A_fn : Constant  Value=21.6
  A_ns : Constant  Value=pi*2.5/2*(2.5+9)
  A_part : Constant  Value=19.62
  A_wd : Constant  Value=2.88
  Add1 : Sum  Inputs=6
  Add2 : Sum  Inputs=3
  Divide : Product  Inputs=***/
  Divide1 : Product  Inputs=***/
  Divide2 : Product  Inputs=4
  Divide3 : Product  Inputs=*/
  Divide4 : Product  Inputs=/*
  Divide5 : Product  Inputs=/*
  Divide6 : Product  Inputs=/*
  MATLAB Function : MATLAB Function  TreatAsAtomicUnit=on
  Mux : Mux  Inputs=7
  Tau_part : Constant  Value=0.5
  Tau_s,wall : Constant  Value=0.89
  k_cork : Constant  Value=0.07
  k_nylon : Constant  Value=0.25
  k_part : Constant  Value=0.49
  k_wool : Constant  Value=0.039
  t_cork : Constant  Value=0.02
  t_nylon : Constant  Value=0.25e-3
  t_part : Constant  Value=0.18
  t_wool : Constant  Value=9.95e-2
  Tin,n : Outport
  wires:
  Divide1/1 -> Add1/6, Divide5/2
  t_wool/1 -> Mux/4
  A_part/1 -> Divide/3
  Divide3/1 -> Add2/3
  Divide5/1 -> Add2/2
  MATLAB Function/1(y) -> Add1/1, Divide3/1
  Tamb/1 -> Mux/6, Divide5/1, Divide3/2, Divide1/2
  Tau_part/1 -> Divide2/4
  Tpart/1 -> Divide4/1, Divide/1
  t_nylon/1 -> Mux/1
  Electrolyzer Heat/1 -> Add1/2
  t_part/1 -> Divide/4
  A_fn/1 -> Divide1/3
  k_nylon/1 -> Mux/2
  Divide2/1 -> Add1/4
  A_wd/1 -> Divide2/2
  Add1/1 -> Divide6/2
  A_ns/1 -> Mux/5
  FC Heat/1 -> Add1/5
  Divide6/1 -> Tin,n/1
  Add2/1 -> Divide6/1
  Divide/1 -> Add1/3, Divide4/2
  k_cork/1 -> Divide1/1
  k_wool/1 -> Mux/3
  k_part/1 -> Divide/2
  Phi/1 -> Mux/7, Divide2/1
  t_cork/1 -> Divide1/4
  Tau_s,wall/1 -> Divide2/3
  Mux/1 -> MATLAB Function/1(u)
  Divide4/1 -> Add2/1

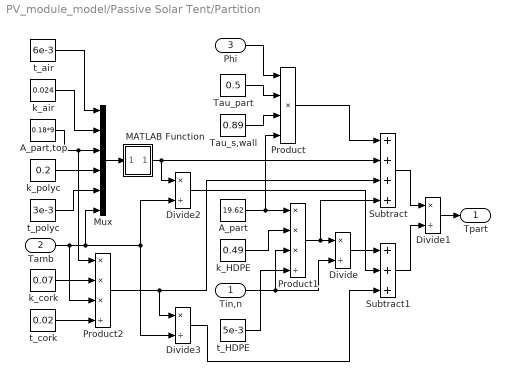
== system PV_module_model/Passive Solar Tent/Partition ==
  Tin,n : Inport
  Tamb : Inport  Port=2
  Phi : Inport  Port=3
  A_part : Constant  Value=19.62
  A_part,top : Constant  Value=0.18*9
  Divide{,1..3} (4 alike) : Product  Inputs=*/
  MATLAB Function : MATLAB Function  TreatAsAtomicUnit=on
  Mux : Mux  Inputs=6
  Product : Product  Inputs=4
  Product1 : Product  Inputs=***/
  Product2 : Product  Inputs=***/
  Subtract : Sum  Inputs=4
  Subtract1 : Sum  Inputs=3
  Tau_part : Constant  Value=0.5
  Tau_s,wall : Constant  Value=0.89
  k_HDPE : Constant  Value=0.49
  k_air : Constant  Value=0.024
  k_cork : Constant  Value=0.07
  k_polyc : Constant  Value=0.2
  t_HDPE : Constant  Value=5e-3
  t_air : Constant  Value=6e-3
  t_cork : Constant  Value=0.02
  t_polyc : Constant  Value=3e-3
  Tpart : Outport
  wires:
  Tau_part/1 -> Product/2
  k_HDPE/1 -> Product1/2
  Tau_s,wall/1 -> Product/3
  Product1/1 -> Subtract/4, Divide/1
  Divide1/1 -> Tpart/1
  Subtract/1 -> Divide1/1
  Phi/1 -> Product/1
  Tin,n/1 -> Divide/2, Product1/3
  A_part/1 -> Product/4, Product1/1
  Product/1 -> Subtract/1
  t_polyc/1 -> Mux/5
  k_air/1 -> Mux/2
  A_part,top/1 -> Product2/1, Mux/3
  k_polyc/1 -> Mux/4
  t_air/1 -> Mux/1
  Mux/1 -> MATLAB Function/1(u)
  Tamb/1 -> Product2/3, Divide3/2, Divide2/2, Mux/6
  t_HDPE/1 -> Product1/4
  t_cork/1 -> Product2/4
  k_cork/1 -> Product2/2
  MATLAB Function/1(y) -> Divide2/1, Subtract/2
  Product2/1 -> Divide3/1, Subtract/3
  Divide/1 -> Subtract1/1
  Divide2/1 -> Subtract1/2
  Divide3/1 -> Subtract1/3
  Subtract1/1 -> Divide1/2

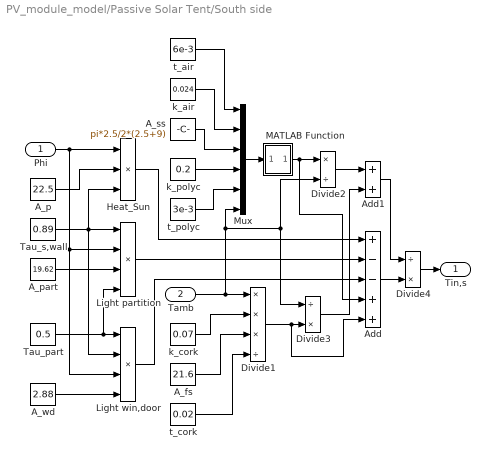
== system PV_module_model/Passive Solar Tent/South side ==
  Phi : Inport
  Tamb : Inport  Port=2
  A_fs : Constant  Value=21.6
  A_p : Constant  Value=22.5
  A_part : Constant  Value=19.62
  A_ss : Constant  Value=pi*2.5/2*(2.5+9)
  A_wd : Constant  Value=2.88
  Add : Sum  Inputs=+--++
  Add1 : Sum
  Divide1 : Product  Inputs=***/
  Divide2 : Product  Inputs=*/
  Divide3 : Product  Inputs=/*
  Divide4 : Product  Inputs=/*
  Heat_Sun : Product  Inputs=3
  Light partition : Product  Inputs=4
  Light win,door : Product  Inputs=4
  MATLAB Function : MATLAB Function  TreatAsAtomicUnit=on
  Mux : Mux  Inputs=6
  Tau_part : Constant  Value=0.5
  Tau_s,wall : Constant  Value=0.89
  k_air : Constant  Value=0.024
  k_cork : Constant  Value=0.07
  k_polyc : Constant  Value=0.2
  t_air : Constant  Value=6e-3
  t_cork : Constant  Value=0.02
  t_polyc : Constant  Value=3e-3
  Tin,s : Outport
  wires:
  Tau_s,wall/1 -> Light win,door/2, Light partition/1, Heat_Sun/3
  Mux/1 -> MATLAB Function/1(u)
  Divide4/1 -> Tin,s/1
  Tau_part/1 -> Light partition/4, Light win,door/1
  A_fs/1 -> Divide1/3
  Tamb/1 -> Divide1/1, Divide3/1, Divide2/2, Mux/6
  Divide1/1 -> Add/5, Divide3/2
  Phi/1 -> Heat_Sun/1, Light partition/2, Light win,door/3
  k_cork/1 -> Divide1/2
  Divide2/1 -> Add1/1
  Heat_Sun/1 -> Add/1
  A_part/1 -> Light partition/3
  Light win,door/1 -> Add/3
  A_wd/1 -> Light win,door/4
  Divide3/1 -> Add1/2
  A_p/1 -> Heat_Sun/2
  Add1/1 -> Divide4/1
  t_cork/1 -> Divide1/4
  Add/1 -> Divide4/2
  Light partition/1 -> Add/2
  t_air/1 -> Mux/1
  k_air/1 -> Mux/2
  A_ss/1 -> Mux/3
  k_polyc/1 -> Mux/4
  t_polyc/1 -> Mux/5
  MATLAB Function/1(y) -> Add/4, Divide2/1

== matlab function PV_module_model/Fuel Cell Final/Fuel Cell/Nernst1 ==
  data: u input; y output
function y = fcn(u)

if u(4) > 0
    u(4) = -u(4);
end
if u(2) > 0
    u(2) = -u(2);
end
if u(3) > 0
    u(3) = -u(3);
end
y = u(1) + u(2) + u(3) + u(4);
u(1);
u(2);
u(3);
u(4);

== matlab function PV_module_model/Fuel Cell Final/Fuel Cell/Vconc ==
  data: u input; y7 output
function y7 = fcn(u)

y7 = u(1)*exp(u(2)*u(3)*10^3);

== matlab function PV_module_model/Fuel Cell Final/Fuel Cell/cH2' ==
  data: u input; y4 output
function y4 = fcn(u)

y4 = (u(1)*9.174*10^-7)*exp(-77/u(2)); %pH2 in atm; cH2 in mol/cm3

== matlab function PV_module_model/Electrolyzer Final/Voltage/C_H2,mem ==
  data: u input; yh output
function yh = fcn(u)

yh = (((u(2)*10^5)*u(3)/(8.314*u(1)))/(10^6)) + (u(6)*u(4)/u(5));

== matlab function PV_module_model/Electrolyzer Final/Voltage/C_O2,mem ==
  data: u input; yo output
function yo = fcn(u)

yo = (((u(2)*10^5)*u(3)/(8.314*u(1)))/(10^6)) + (u(6)*u(4)/u(5));

== matlab function PV_module_model/Electrolyzer Final/Voltage/Eo ==
  data: u input; y output
function y = fcn(u)

y = 1.229 - 0.85*(10^-3)*(u - 298);

== matlab function PV_module_model/Electrolyzer Final/Voltage/Vact ==
  data: u input; y output
function y = fcn(u)

y = ((8.314*u(1)/(u(2)*96485))*asinh(u(3)/(2*u(4)))) + ((8.314*u(1)/(u(5)*96485))*asinh(u(3)/(2*u(6))));

== matlab function PV_module_model/Electrolyzer Final/Voltage/Vcon,an ==
  data: u input; y output
function y = fcn(u)
if u(3) < 0
    u(3) = -u(3);
end
y = (8.314*u(1)/(4*96485))*log(u(3)/u(2));

== matlab function PV_module_model/Electrolyzer Final/Voltage/Vcon,cat ==
  data: u input; y output
function y = fcn(u)
if u(3) < 0
    u(3) = -u(3);
end
y = (8.314*u(1)/(2*96485))*log(u(3)/u(2));

== matlab function PV_module_model/Electrolyzer Final/Effective Diffusion/Deff H2O,K ==
  data: u input; y1 output
function y1 = fcn(u)

y1 = ((4/3)*(1*10^-6)*sqrt((8*8.314*u)/(pi*18/1000)))*10^4; % 10^4 is to convert m2/s to cm2/s

== matlab function PV_module_model/Electrolyzer Final/Voltage/Voc ==
  data: u input; y output
function y = fcn(u)
u(1);
u(2);
if u(1) < 0
    u(1) = -u(1);
end
if u(2) < 0
    u(2) = -u(2);
end

y = u(4) + (8.314*u(3)/(2*96485))*log(u(2)*(u(1)^0.5));

== matlab function PV_module_model/Electrolyzer Final/Voltage/sigma_mem ==
  data: u input; y output
function y = fcn(u)

y = (0.005139*u(2) - 0.00326)*exp(1268*((1/303) - (1/u(1))));

== matlab function PV_module_model/Fuel Cell Final/Fuel Cell/cO2' ==
  data: u input; y3 output
function y3 = fcn(u)

y3 = (u(1)*1.97*10^-7)*exp(498/u(2)); %pO2 in atm, cO2 in mol/cm3

== matlab function PV_module_model/Fuel Cell Final/Fuel Cell/rM ==
  data: u input; y6 output
function y6 = fcn(u)

y6 = (181.6*(1 + 0.03*(u(1)/u(4)) + 0.062*((u(2)/303)^2)*((u(1)/u(4))^2)))/((u(3) - 0.634 - 3*(u(1)/u(4)))*exp(4.18*(u(2)-303)/u(2)));

== matlab function PV_module_model/MATLAB Function ==
  data: u input; y output
function y = fcn(u)

if u < 100
    y = 100;
else 
    y = u;
end

== matlab function PV_module_model/MATLAB Function1 ==
  data: u input; y output
function y = fcn(u)

if u < 40
    y = 1;
else 
    y = u;
end

== matlab function PV_module_model/Solar PV efficiency ==
  data: u input; eff output
function eff = fcn(u)
% u(1) is Irradiance input, u(2) is solar PV output

if u(2) > 1
    eff = u(2)/(2*u(1))*100;           %area of module included as 2 in denominator
else
    eff = 0;
end

== matlab function PV_module_model/N_Electrolyzers ==
  data: u input; y output
function y = fcn(u)


if u <= 400
    y = u;

elseif (400 < u)&&(u <= 800)
    y = u/2;

elseif (800 < u)&&(u <= 1200)
    y = u/3;

elseif (1200 < u)&&(u <= 1600)
    y = u/4;

else 
    y = u/5;
end

== matlab function PV_module_model/N_Electrolyzers  ==
  data: u input; NH2 output; NO2 output
function [NH2,NO2] = fcn(u)
% u(1) is input power, u(2) is NH2, u(3) is NO2

if u(1) <= 400
    NH2 = u(2);
    NO2 = u(3);

elseif (400 < u(1))&&(u(1) <= 800)
    NH2 = u(2)*2;
    NO2 = u(3)*2;

elseif (800 < u(1))&&(u(1) <= 1200)
    NH2 = u(2)*3;
    NO2 = u(3)*3;

elseif (1200 < u(1))&&(u(1) <= 1600)
    NH2 = u(2)*4;
    NO2 = u(3)*4;

else 
    NH2 = u(2)*5;
    NO2 = u(3)*5;
end

== matlab function PV_module_model/Passive Solar Tent/North side/MATLAB Function ==
  data: u input; y output
function y = fcn(u)

y = (u(5)*u(6))/(4*((2*u(1)/u(2)) + (u(4)/u(3))));

== matlab function PV_module_model/Electrolyzer Final/Effective Diffusion/Deff O2-H2O ==
  data: u input; y3 output
function y3 = fcn(u)

y3 = (0.00133*(((1/32) + (1/18))^0.5)*((u(2)^1.5)/(u(1)*(u(4)^2)*u(3))))*10^4;

== matlab function PV_module_model/Passive Solar Tent/Partition/MATLAB Function ==
  data: u input; y output
function y = fcn(u)

y = (u(3)*u(6))/((2*u(5)/u(4)) + (u(1)/u(2)));

== matlab function PV_module_model/Passive Solar Tent/South side/MATLAB Function ==
  data: u input; y output
function y = fcn(u)

y = (u(3)*u(6))/((2*u(5)/u(4)) + (u(1)/u(2)));

== matlab function PV_module_model/Electrolyzer efficiency ==
  data: u input; heat output; eff output
function [heat,eff] = fcn(u)
%u(1) is NH2, u(2) is input power, u(3) is H2 HHV

if u(2) > 1
    heat = u(2) - u(1)*u(3);
else
    heat = 0;
end


if u(2) > 1
    eff = u(1)*u(3)/u(2)*100;
else
    eff = 0;
end

== matlab function PV_module_model/Electrolyzer Input Power ==
  data: u input; y output
function y = fcn(u)
%u(1) is load, u(2) is power input from solar PV

if u(1) <= u(2)
    y = u(2) - u(1);
else
    y = 1;
end

== matlab function PV_module_model/FC Power  ==
  data: u input; y output
function y = fcn(u)
%u(1) is solar power, u(2) is load, u(3) is fuel cell power

if u(1) < u(2)
    y = u(3);
else
    y = 0;
end

== matlab function PV_module_model/FC efficiency ==
  data: u input; heat output; eff output
function [heat,eff] = fcn(u)
%u(1) is FC Power output, u(2) is m.H2used, u(3) is H2 HHV

if u(2) > 0
    heat = u(2)*u(3) - u(1);
else
    heat = 0;
end


if u(2) > 0
    eff = u(1)/(u(2)*u(3))*100;
else
    eff = 0;
end

== matlab function PV_module_model/Load req ==
  data: u input; y output
function y = fcn(u)
%u(1) is load, u(2) is power input from solar PV

if u(1) > u(2)
    y = u(1) - u(2)
else
    y = 0.000001;
end

== matlab function PV_module_model/Solar PV final/Imp ==
  data: u input; y output
function y = fcn(u)
iold = u(4)-0.05;
inew = 9;

for i = 1:500  
    inew = iold - ((u(3)*((iold/(iold - u(4) - u(2))) + log((u(4) - iold + u(2))/u(2))) - 2*iold*u(1))/(u(3)*((iold - 2*u(4) - 2*u(2))/((iold - u(4) - u(2))^2)) - 2*u(1)));
    %i_inter = inew - (u(3)*log(10^12))/(u(3)*((i - 2*u(4) - 2*u(2))/((i - u(4) - u(2))^2)) - 2*u(1)); 
    iold = inew;

end
y = inew;
end

== matlab function PV_module_model/Solar PV final/Io ==
  data: u input; y output
function y = fcn(u)

y = u(2)*((u(5)/u(4))^3)*exp(u(3)*1.6*(10^-19)*u(6)*(1-(u(5)/u(4)))/(u(1)*1.6*10^-19));

== matlab function PV_module_model/Electrolyzer Final/Effective Diffusion/Deff_an ==
  data: u input; y2 output
function y2 = fcn(u)

y2 = 1/((0.3/4)*((1/u(1)) + (1/(u(2)))));

== matlab function PV_module_model/Solar PV final/Io,ref ==
  data: u input; y output
function y = fcn(u)

y = u(3)*exp(-u(2)/u(1));

== matlab function PV_module_model/Solar PV final/Isc ==
  data: u input; y output
function y = fcn(u)

y = (u(4)/u(5))*(u(1) + u(6)*(u(2) - u(3)));

== matlab function PV_module_model/Solar PV final/Rs ==
  data: u input; y output
function y = fcn(u)

y = ((u(5)*log(1-(u(1)/u(4)))) + u(3) - u(2))/u(1);

== matlab function PV_module_model/Solar PV final/Vmp ==
  data: u input; y output
function y = fcn(u)

y = (u(4)*log(((u(5) - u(3))/u(2)) + 1)) - u(3)*u(1);

== matlab function PV_module_model/Solar PV final/alpha,ref ==
  data: u input; y output
function y = fcn(u)

y = ((2*u(1) - u(3))/((u(4)/(u(4)-u(2))) + log(1-(u(2)/u(4)))));

== matlab function PV_module_model/m.H2 real ==
  data: u input; y output
function y= fcn(u)
%u(1) is solar power, u(2) is load, u(3) is m.H2 fuel cell

if u(1) < u(2)
    y = u(3);
else
    y = 0;
end

== matlab function PV_module_model/Electrolyzer Final/Effective Diffusion/Deff_cat ==
  data: u input; y1 output
function y1 = fcn(u)

y1 = 1/((0.3/4)*((1/u(1)) + (1/(u(2)))));

== matlab function PV_module_model/Electrolyzer Final/Effective Diffusion/eps//k H2-H2O ==
  data: u input; y output
function y = fcn(u)

y = sqrt(u(1)*u(2));

== matlab function PV_module_model/Electrolyzer Final/Effective Diffusion/eps//k O2-H2O ==
  data: u input; y output
function y = fcn(u)

y = sqrt(u(1)*u(2));

== matlab function PV_module_model/Electrolyzer Final/Effective Diffusion/omegaD H2-H2O ==
  data: u input; y5 output
function y5 = fcn(u)

y5 = (1.06036/(u^0.1561)) + (0.193/exp(0.47635*u)) + (1.03587/exp(1.52996*u)) + (1.76474/(3.89411*u));

== matlab function PV_module_model/Electrolyzer Final/Effective Diffusion/omegaD O2-H2O ==
  data: u input; y4 output
function y4 = fcn(u)

y4 = (1.06036/(u^0.1561)) + (0.193/exp(0.47635*u)) + (1.03587/exp(1.52996*u)) + (1.76474/(3.89411*u));

== matlab function PV_module_model/Electrolyzer Final/Membrane/MATLAB Function ==
  data: data1 input; u input; y output; data input
function y = fcn(data1, u, data)
data1;
u;
data;
y = data1 - u + data;

== matlab function PV_module_model/Fuel Cell Final/Fuel Cell/Eo ==
  data: u input; y1 output
function y1 = fcn(u)

y1 = 1.229 - 0.85*10^-3*(u-298.15);

== matlab function PV_module_model/Fuel Cell Final/Fuel Cell/Eta__act ==
  data: u input; y5 output
function y5 = fcn(u)

if u(4) <0
    u(4) = -u(4);
end
if u(2) <0
    u(2) = -u(2);
end
if u(3) <0
    u(3) = -u(3);
end
if u(5) <0
    u(5) = -u(5);
end

y5 = (-0.948) + ((0.00286 + 0.0002*log(u(4)) + 4.3*10^-5*log(u(2)))*u(1)) + (u(1)*log(u(3))*7.6*10^-5) - (u(1)*log(u(5))*1.93*10^-4); %replace log(0.11) by log(u(5)

u(5);

== matlab function PV_module_model/Electrolyzer Final/Effective Diffusion/Deff H2-H2O ==
  data: u input; y2 output
function y2 = fcn(u)

y2 = (0.00133*(((1/2) + (1/18))^0.5)*((u(2)^1.5)/(u(1)*(u(4)^2)*u(3))))*10^4; %10^4 is for m2/s to cm2/s

== matlab function PV_module_model/Fuel Cell Final/Fuel Cell/Nernst ==
  data: u input; y2 output
function y2 = fcn(u)

if u(4) < 0
    u(4) = -u(4);
end
if u(5) <0
    u(5) = -u(5);
end

y2 = (u(1)*u(2)/(2*u(3)))*log(u(4)*(u(5)^0.5));
